simulink model "simulator"  (R2023a)
settings: Solver=VariableStepAuto  StartTime=0.0  StopTime=50  FixedStep=1/60  MinStep=1/60  RelTol=1e-3
values from neighbouring files (symbols this model uses):
  y0 = -45    [generate_runner_trajectory.m]    (also in steering_controller.m = b * rho)
libraries: sim3dlib x5, visionsinks x3, vdynlib x2
settings Model: Creator=jonasoba  LastModifiedBy=jonasoba

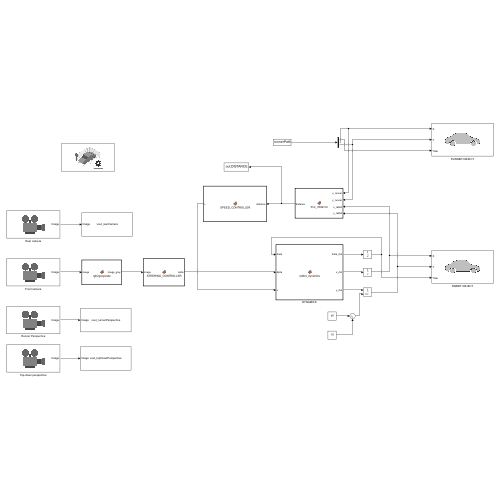
[thumbnail: Simulink's stored preview of the top-level diagram]
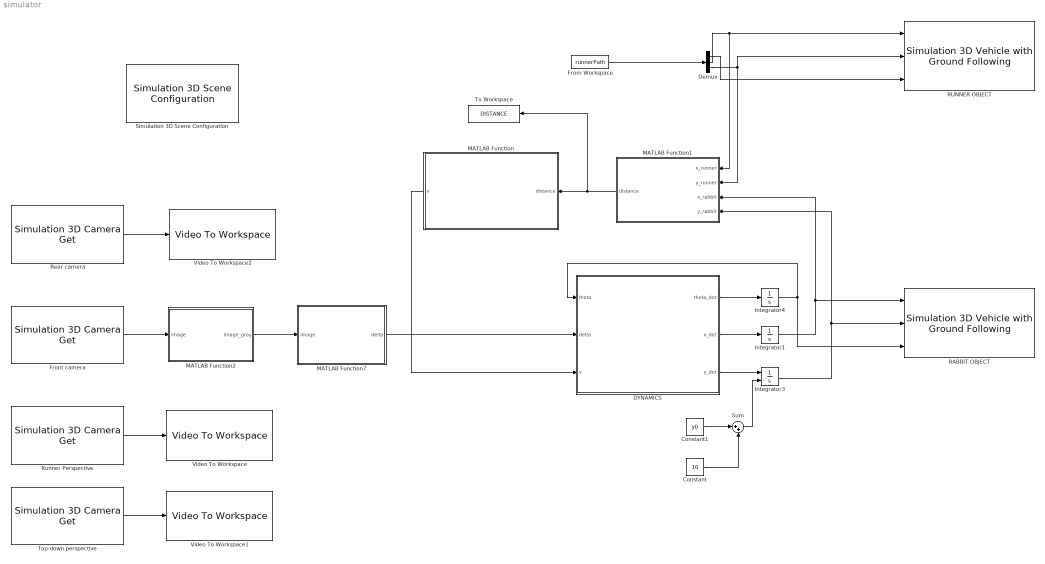
== system simulator ==
  Constant : Constant  Value=10
  Constant1 : Constant  Value=y0
  DYNAMICS : MATLAB Function  TreatAsAtomicUnit=on
  Demux : Demux  Outputs=3
  From Workspace : FromWorkspace  VariableName=runnerPath
  Front camera : sim3dlib/Simulation 3D Camera Get  Priority=1  sensorTag=Sim3dSensor1  sensorId=1  sensorName=Sim3dSensor1  vehTagList={'Scene Origin';'hare';'muscleboy'}  vehTag=hare  mountLoc=Front bumper  offsetFlag=on  tmountOffset=[0, 1, 0]  rmountOffset=[0, 20, 0]  HorizontalResolution=1280  VerticalResolution=720  HorizontalFOV=80  SampleTime=-1  mountPoint=[1.29999995231628 -1 0.300000011920929]  mountOrientation=[0 -20 0]  aMode=5  ID=1
      settings: LibrarySourceBlock=sl3dlib/Simulation 3D/Simulation 3D Camera Get
  Integrator1 : Integrator  InitialCondition=-39.55
  Integrator3 : Integrator  InitialConditionSource=external  InitialCondition=-45
  Integrator4 : Integrator  InitialCondition=pi/2+0.2
  MATLAB Function : MATLAB Function  TreatAsAtomicUnit=on
  MATLAB Function1 : MATLAB Function  TreatAsAtomicUnit=on
  MATLAB Function2 : MATLAB Function  TreatAsAtomicUnit=on
  MATLAB Function7 : MATLAB Function  TreatAsAtomicUnit=on
  RABBIT OBJECT : vdynlib/Vehicle Scenarios/Sim3D/Sim3D Vehicle/Components/Simulation 3D Vehicle with Ground Following  Priority=-1  PassVehMesh=Formula student vehicle  MeshPath=/MathWorksSimulation/Vehicles/Muscle/Meshes/SK_MuscleCar.SK_MuscleCar  TrackWidth=1.9  WheelBase=3  WheelRadius=0.35  VehColor=Green  InitialPos=[0, 0, 0]  InitialRot=[0, 0, 0]  ActorName=hare  VehLightsControl=off  HeadlightColor=[ 1, 1, 1 ]  HighBeamIntensity=100000  LowBeamIntensity=60000  HighBeamConeAngle=1.22  LowBeamConeAngle=1.22  LeftHeadlightOrientation=[ 0, 0 ]  RightHeadlightOrientation=[ 0, 0 ]  BrakelightIntensity=200  ReverselightIntensity=500  SignallightIntensity=500  SignallightPeriod=1  SignalPulseWidth=50  SampleTime=-1  ActorType=SimulinkVehicle  ID=C  aMode=2  ActorTag=hare  CoordinateScheme=SAE
  RUNNER OBJECT : vdynlib/Vehicle Scenarios/Sim3D/Sim3D Vehicle/Components/Simulation 3D Vehicle with Ground Following  Priority=-1  PassVehMesh=Box truck  MeshPath=/MathWorksSimulation/Vehicles/Muscle/Meshes/SK_MuscleCar.SK_MuscleCar  TrackWidth=1.9  WheelBase=3  WheelRadius=0.35  VehColor=Red  InitialPos=[0, 0, 0]  InitialRot=[0, 0, 0]  ActorName=muscleboy  VehLightsControl=off  HeadlightColor=[ 1, 1, 1 ]  HighBeamIntensity=100000  LowBeamIntensity=60000  HighBeamConeAngle=1.22  LowBeamConeAngle=1.22  LeftHeadlightOrientation=[ 0, 0 ]  RightHeadlightOrientation=[ 0, 0 ]  BrakelightIntensity=200  ReverselightIntensity=500  SignallightIntensity=500  SignallightPeriod=1  SignalPulseWidth=50  SampleTime=-1  ActorType=SimulinkVehicle  ID=C  aMode=2  ActorTag=muscleboy  CoordinateScheme=SAE
  Rear camera : sim3dlib/Simulation 3D Camera Get  Priority=1  sensorTag=Sim3dSensor4  sensorId=4  sensorName=Sim3dSensor4  vehTagList={'Scene Origin';'hare';'muscleboy'}  vehTag=hare  mountLoc=Rear bumper  offsetFlag=on  tmountOffset=[0, 1, 0]  rmountOffset=[0, 0, 0]  HorizontalResolution=640  VerticalResolution=480  HorizontalFOV=60  SampleTime=-1  mountPoint=[-1.39999997615814 -1 0.300000011920929]  mountOrientation=[0 0 180]  aMode=5  ID=4
      settings: LibrarySourceBlock=sl3dlib/Simulation 3D/Simulation 3D Camera Get
  Runner Perspective : sim3dlib/Simulation 3D Camera Get  Priority=1  sensorTag=Sim3dSensor2  sensorId=2  sensorName=Sim3dSensor2  vehTagList={'Scene Origin';'hare';'muscleboy'}  vehTag=muscleboy  mountLoc=Hood center  offsetFlag=on  tmountOffset=[0, 0, 0]  rmountOffset=[0, 20, 0]  HorizontalResolution=640  VerticalResolution=480  HorizontalFOV=60  SampleTime=-1  mountPoint=[3.79999995231628 0 2.09999990463257]  mountOrientation=[0 -20 0]  aMode=5  ID=2
      settings: LibrarySourceBlock=sl3dlib/Simulation 3D/Simulation 3D Camera Get
  Simulation 3D Scene Configuration : sim3dlib/Simulation 3D Scene Configuration  Priority=0  ProjectFormat=Unreal Editor  SceneDesc=Empty scene  ProjectName=C:\Users\jonasoba\OneDrive - NTNU\MATLAB\Master project\executables\Windows\AutonomHare.exe  ScenePath=/Game/runningTrack_mountains  UEProjPath=C:\project\AutoVrtlEnv\AutoVrtlEnv.uproject  EnableOpenDRIVE=off  vehTagList={'Scene Origin';'hare';'muscleboy'}  vehTag=Scene Origin  OpVisEn=off  Ts=.02  EnableWindow=on  EnableRemoteAccess=off  EnableWeather=off  SunAltitude=40.0  SunAzimuth=90  clouds=10  wind=1  fog=0  rain=0  EnableGeospatial=off  OriginHeight=200  OriginLatitude=40.744652  OriginLongitude=-73.988864  MapStyle=Aerial  AdditionalAssetIDs=[]  UseAdvancedSunSky=off  SolarTime=11  TimeZone=-5  Day=21  Month=9  Year=2022  UseDaylightSavingTime=on  DSTStartDay=10  DSTStartMonth=3  DSTEndDay=3  DSTEndMonth=11  DSTSwitchHour=2  sensorTag=MainCamera2  sensorId=2  sensorName=MainCamera2  mountLoc=Origin  offsetFlag=off  tmountOffset=[0, 0, 0]  rmountOffset=[0, 0, 0]  HorizontalResolution=1280  VerticalResolution=720  HorizontalFOV=60  mountPoint=[0 0 0]  mountOrientation=[0 0 0]  aMode=5  ID=2  GeoTrigger=Inactive
      settings: LibrarySourceBlock=sl3dlib/Simulation 3D/Simulation 3D Scene Configuration
  Sum : Sum  Inputs=|++
  To Workspace : ToWorkspace  VariableName=DISTANCE  SampleTime=-1
  Top-down perspective : sim3dlib/Simulation 3D Camera Get  Priority=1  sensorTag=Sim3dSensor3  sensorId=3  sensorName=Sim3dSensor3  vehTagList={'Scene Origin';'hare';'muscleboy'}  vehTag=muscleboy  mountLoc=Front bumper  offsetFlag=on  tmountOffset=[0, 0, 30]  rmountOffset=[0, 90, 0]  HorizontalResolution=640  VerticalResolution=480  HorizontalFOV=60  SampleTime=-1  mountPoint=[5.09999990463257 0 30.6000003814697]  mountOrientation=[0 -90 0]  aMode=2  ID=3
      settings: LibrarySourceBlock=vdynlib/Vehicle Scenarios/Sim3D/Sim3D Core/Simulation 3D Camera Get
  Video To Workspace : visionsinks/Video To Workspace  VariableName=vout_runnerPerspective  NumInputs=1  DataLimit=inf  DecimationFactor=1  LogFi=off  InPortLabels=R|G|B
  Video To Workspace1 : visionsinks/Video To Workspace  VariableName=vout_topDownPerspective  NumInputs=1  DataLimit=inf  DecimationFactor=1  LogFi=off  InPortLabels=R|G|B
  Video To Workspace2 : visionsinks/Video To Workspace  VariableName=vout_rearCamera  NumInputs=1  DataLimit=inf  DecimationFactor=1  LogFi=off  InPortLabels=R|G|B
  wires:
  From Workspace/1 -> Demux/1
  Demux/3 -> MATLAB Function1/2(y_runner), RUNNER OBJECT/2
  Demux/2 -> MATLAB Function1/1(x_runner), RUNNER OBJECT/1
  Demux/1 -> RUNNER OBJECT/3
  Integrator1/1 -> MATLAB Function1/3(x_rabbit), RABBIT OBJECT/1
  Integrator4/1 -> DYNAMICS/1(theta), RABBIT OBJECT/3
  DYNAMICS/3(y_dot) -> Integrator3/1
  Integrator3/1 -> MATLAB Function1/4(y_rabbit), RABBIT OBJECT/2
  DYNAMICS/2(x_dot) -> Integrator1/1
  DYNAMICS/1(theta_dot) -> Integrator4/1
  Top-down perspective/1 -> Video To Workspace1/1
  MATLAB Function7/1(delta) -> DYNAMICS/2(delta)
  Constant/1 -> Sum/2
  Sum/1 -> Integrator3/2
  Constant1/1 -> Sum/1
  Runner Perspective/1 -> Video To Workspace/1
  MATLAB Function/1(v) -> DYNAMICS/3(v)
  Front camera/1 -> MATLAB Function2/1(image)
  MATLAB Function2/1(image_gray) -> MATLAB Function7/1(image)
  MATLAB Function1/1(distance) -> To Workspace/1, MATLAB Function/1(distance)
  Rear camera/1 -> Video To Workspace2/1

== matlab function simulator/DYNAMICS ==
  data: theta_dot output; x_dot output; theta input; delta input; v input; y_dot output
function [theta_dot, x_dot, y_dot] = rabbit_dynamics(theta, delta, v)
    % Input:
    % - theta:
    % - delta:
    % - v: 
    % Output:
    % - dxdt: time derivatives 


    L = 1;  % Length of the rabbit
    l_r = 0.7;
    % Calculate the time derivatives
    beta = atan2(l_r*tan(delta), L);

    x_dot = v*cos(beta + theta);
    y_dot = v*sin(beta + theta);
    theta_dot = v*tan(delta)*cos(beta)/L;
end

== matlab function simulator/MATLAB Function ==
  data: distance input; v output
function v = SPEED_CONTROLLER(distance)

coder.extrinsic("speed_controller");
v = 1.1; %Helt random verdi for å initialisere og si at det er en double. 

v = speed_controller(distance);

== matlab function simulator/MATLAB Function1 ==
  data: x_runner input; y_runner input; x_rabbit input; distance output; y_rabbit input
function distance = true_distance(x_runner, y_runner, x_rabbit, y_rabbit)

distance = sqrt((x_rabbit-x_runner)^2 + (y_rabbit-y_runner)^2);

== matlab function simulator/MATLAB Function2 ==
  data: image input; image_gray output
function image_gray  = rgb2grayscale(image)


image_gray = rgb2gray(image);



end

== matlab function simulator/MATLAB Function7 ==
  data: image input; delta output
function delta    = STEERING_CONTROLLER(image)

coder.extrinsic("steering_controller");
delta = 1.1; %Helt random verdi for å initialisere og si at det er en double. 

delta = steering_controller(image);

end
